simulink model "ConfiguredVirtualVehicleModel"  (R2023a)
settings: configuration reference "VehicleVariable" (kept outside this file)
StartFcn:
  | %tic
StopFcn:
  | %toc
undefined symbols (not defined in the file or in its folder): CtrlTcuInitGear, CtrlVcuCltch1InitCmd, Disabled, DriveCycleChoice, DriverPreviewDist, EnvAbsPrs, EnvAirTemp, EnvGrvty, EnvNomFrictionScaling, EnvNominalGrade, EnvWindVelX, EnvWindVelY, EnvWindVelZ, FTP75, PlntBattModNumCellSer, PlntBattNumMod, PlntBattTempInitDegC, PlntVehDstCGFrntAxl, PlntVehDstCGRearAxl, PlntVehInitLatPos, PlntVehInitLongPos, PlntVehInitPitchAng, PlntVehInitRollAng, PlntVehInitVertPos, PlntVehInitYawAng, PlntVehMass, PlntVehTrckWdth, PlntVehYawMomentInertia, ScnCRMaxLatAccel, ScnCRRadius, ScnDLCGateLongPos, ScnDLCLatRef, ScnDLCLatRefOffset, ScnDLCLongRefBpt, ScnDLCLongRefStartPos, ScnDLCVehicleWidth, ScnFHCounterDwellTime, ScnFHInitialDwellTime, ScnFHReturnTime, ScnFHRollRateZeroCross, ScnFHSteerAmp, ScnFHSteerSpeed, ScnISHandwheelRate, ScnISMaxHandwheelAng, ScnISMaxLatAccel, ScnISSteerHoldTime, ScnLongVelRef, ScnSDDwellTime, ScnSDSteerAmp, ScnSDSteerFreq, ScnSimTime, ScnSSFinalFreq, ScnSSSteerAmp, ScnSSSweepTime, ScnStartTime, ts
libraries: simulink x18, vehdynlibscenariocommon x7, autolibshared x5, vehdynlibviscommon x3, vehdynlibdriver x2, sim3dgroundtruthsensorlib x2, autolibsharedcommon x1, sharedtransform x1, sim3dlib x1, sim3dautolib x1
(part 4 of 5)

== system ConfiguredVirtualVehicleModel/Visualization/Vehicle XY Plotter/XY View Ref ==
  Bus Element In2 : Inport  PortName=VehFdbk
  Bus Element In1 : Inport  Port=2  PortName=Ref  Element=YRef
  Bus Element In3 : Inport  Port=2  PortName=Ref  Element=XRef
  Bus Selector1 : BusSelector  OutputSignals=Body.InertFrm.Cg.Ang.phi,Body.InertFrm.Cg.Ang.theta,Body.InertFrm.Cg.Ang.psi  OutputAsBus=on
  Bus Selector10 : BusSelector  OutputSignals=Wheels.Wheels.Fx,Wheels.Wheels.Fy
  Bus Selector5 : BusSelector  OutputSignals=Steering.Front.WhlAng.FL,Steering.Front.WhlAng.FR,Steering.Rear.WhlAng.RL,Steering.Rear.WhlAng.RR  OutputAsBus=on
  Bus Selector6 : BusSelector  OutputSignals=Body.InertFrm.Geom.Disp.X,Body.InertFrm.Geom.Disp.Y,Body.InertFrm.Geom.Disp.Z  OutputAsBus=on
  Bus Selector7 : BusSelector  OutputSignals=Body.InertFrm.Geom.Vel.Xdot,Body.InertFrm.Geom.Vel.Ydot,Body.InertFrm.Geom.Vel.Zdot  OutputAsBus=on
  Bus Selector9 : BusSelector  OutputSignals=Driveline.EngSpd,Driveline.TransInfo.TransInfo.Trans.TransGear  OutputAsBus=on
  Bus to Vector{,1..3} (4 alike) : BusToVector
  Ground1 : Ground
  Mux : Mux  Inputs=3
  Vehicle XY Plotter : vehdynlibviscommon/Vehicle XY Plot Configuration  extRef=on  extStats=on  extTireF=on  a=PlntVehDstCGFrntAxl  b=PlntVehDstCGRearAxl  w=PlntVehTrckWdth(1)  figBorder=10  bufferSize=1024  velNorm=5  tireFNorm=1000  pltDT=.1
  wires:
  Bus Selector7/1 -> Bus to Vector1/1
  Bus Selector5/1 -> Vehicle XY Plotter/4
  Ground1/1 -> Mux/3
  Bus Selector10/2 -> Vehicle XY Plotter/8  "<Fy>"
  Bus to Vector1/1 -> Vehicle XY Plotter/3
  Bus Selector10/1 -> Vehicle XY Plotter/7  "<Fx>"
  Bus Selector1/1 -> Bus to Vector2/1
  Bus Selector9/1 -> Bus to Vector3/1
  Bus Element In1/1 -> Mux/2
  Bus to Vector3/1 -> Vehicle XY Plotter/6
  Bus Element In3/1 -> Mux/1
  Mux/1 -> Vehicle XY Plotter/5
  Bus to Vector/1 -> Vehicle XY Plotter/1
  Bus Selector6/1 -> Bus to Vector/1
  Bus to Vector2/1 -> Vehicle XY Plotter/2
  Bus Element In2/1 -> Bus Selector10/1, Bus Selector9/1, Bus Selector5/1, Bus Selector7/1, Bus Selector1/1, Bus Selector6/1  "VehFdbk"

== system ConfiguredVirtualVehicleModel/Driver Commands/Driver Commands/Longitudinal Driver/Hill Hold ==
  LngRef : Inport
  <EnblDecelCmd> : Inport  Port=2
  <DecelOvrCmd> : Inport  Port=3
  <DecelHld> : Inport  Port=4
  <DecelZero> : Inport  Port=5
  Env : Inport  Port=6
  VehFdbk : Inport  Port=7
  Abs : Abs  ZeroCross=off  SaturateOnIntegerOverflow=off
  Abs1 : Abs  ZeroCross=off  SaturateOnIntegerOverflow=off
  Bus Selector : BusSelector  OutputSignals=Engine.EngSpdOut,Body.BdyFrm.Cg.Vel.xdot,Battery.BattSoc
  Bus Selector1 : BusSelector  OutputSignals=Body.BdyFrm.Cg.Vel.xdot
  Bus Selector2 : BusSelector  OutputSignals=Grade
  Compare To Constant : simulink/Logic and Bit Operations/Compare To Constant  relop=<=  const=.1  OutDataTypeStr=boolean  ZeroCross=off
  Compare To Constant1 : simulink/Logic and Bit Operations/Compare To Constant  relop=>=  const=.1  OutDataTypeStr=boolean  ZeroCross=off
  Compare To Constant2 : simulink/Logic and Bit Operations/Compare To Constant  relop=<=  const=500  OutDataTypeStr=boolean  ZeroCross=off
  Compare To Constant3 : simulink/Logic and Bit Operations/Compare To Constant  relop=<=  const=5  OutDataTypeStr=boolean  ZeroCross=off
  Compare To Constant4 : simulink/Logic and Bit Operations/Compare To Constant  relop=<=  const=.1  OutDataTypeStr=boolean  ZeroCross=off
  Data Type Conversion1 : DataTypeConversion  SaturateOnIntegerOverflow=off  RndMeth=Floor
  Igore Initialization Transients (t<=2s) : Subsystem
  Logical Operator : Logic  AllPortsSameDT=off  OutDataTypeStr=boolean
  Logical Operator1 : Logic  Inputs=3  AllPortsSameDT=off  OutDataTypeStr=boolean
  Logical Operator2 : Logic  Operator=OR  AllPortsSameDT=off  OutDataTypeStr=boolean
  Signal Specification : SignalSpecification  Unit=m/s
  Switch : Switch  Criteria=u2 > Threshold  SaturateOnIntegerOverflow=off  InputSameDT=off
  Switch1 : Switch  Criteria=u2 > Threshold  SaturateOnIntegerOverflow=off  InputSameDT=off
  Unit Conversion : UnitConversion
  VehFdbk1 : InportShadow  Port=7
  EnblDecelOvr : Outport
  DecelOvrCmd : Outport  Port=2
  DecelHld : Outport  Port=3
  DecelZero : Outport  Port=4
  VelFdbk : Outport  Port=5
  Grade : Outport  Port=6
  wires:
  Logical Operator2/1 -> Switch/3, Data Type Conversion1/1
  LngRef/1 -> Abs/1
  Abs/1 -> Compare To Constant/1
  Compare To Constant/1 -> Logical Operator/1
  Abs1/1 -> Compare To Constant1/1
  Compare To Constant1/1 -> Logical Operator/2
  Compare To Constant2/1 -> Logical Operator1/1
  Compare To Constant3/1 -> Logical Operator1/2
  Logical Operator1/1 -> Logical Operator2/1
  Logical Operator/1 -> Logical Operator2/2
  Compare To Constant4/1 -> Logical Operator1/3
  VehFdbk/1 -> Bus Selector/1
  Bus Selector/1 -> Compare To Constant2/1  "<EngSpdOut>"
  Bus Selector/2 -> Unit Conversion/1  "<xdot>"
  Bus Selector/3 -> Compare To Constant4/1  "<BattSoc>"
  Data Type Conversion1/1 -> Switch1/3
  <EnblDecelCmd>/1 -> Switch1/2, Switch/1, Switch/2
  Switch/1 -> EnblDecelOvr/1
  <DecelOvrCmd>/1 -> Switch1/1
  Switch1/1 -> DecelOvrCmd/1
  Env/1 -> Bus Selector2/1
  Bus Selector2/1 -> Grade/1, Abs1/1  "<Grade>"
  VehFdbk1/1 -> Bus Selector1/1
  Bus Selector1/1 -> Igore Initialization Transients (t<=2s)/1(<xdot>)  "<xdot>"
  Igore Initialization Transients (t<=2s)/1(VelFdbk) -> VelFdbk/1
  <DecelZero>/1 -> DecelZero/1
  <DecelHld>/1 -> DecelHld/1
  Unit Conversion/1 -> Signal Specification/1
  Signal Specification/1 -> Compare To Constant3/1

== system ConfiguredVirtualVehicleModel/Driver Commands/Driver Commands/Longitudinal Driver/Longitudinal Driver ==
  VelRef : Inport  Unit=m/s
  EnblAccelOvr : Inport  Port=2
  AccelOvrCmd : Inport  Port=3
  AccelHld : Inport  Port=4
  AccelZero : Inport  Port=5
  EnblDecelOvr : Inport  Port=6
  DecelOvrCmd : Inport  Port=7
  DecelHld : Inport  Port=8
  DecelZero : Inport  Port=9
  VelFdbk : Inport  Port=10  Unit=m/s
  Grade : Inport  Port=11
  ExtGearGround : Ground
  External Action Routing : Subsystem
  Longitudinal Driver : autolibsharedcommon/Longitudinal Driver  cntrlType=Predictive  shftType=None  vnom=vnom  Kp=Kp  Ki=Ki  Kaw=Kaw  Kff=Kff  Kg=Kg  tauerr=tauerr  tShift=tShift  tRev=tRev  tPark=tPark  pdlVec=pdlVec  upShftTbl=upShftTbl  dwnShftTbl=dwnShftTbl  GearInit=GearInit  tClutch=tClutch  VehVelVec=VehVelVec  KffVec=KffVec  KiVec=KiVec  KpVec=KpVec  KgVec=KgVec  m=m  Kpt=Kpt  Lvv=L  g=g  UpGearVec=UpGearVec  DownGearVec=DownGearVec  aMode=6  errUnit=m/s  aR=aR  bR=bR  cR=cR  tauPt=tauPt
      settings: LibrarySourceBlock=autolibshared/Longitudinal Driver/Longitudinal Driver
  Info : Outport  InitialOutput=0  VectorParamsAs1DForOutWhenUnconnected=off
  AccelCmd : Outport  Port=2  VectorParamsAs1DForOutWhenUnconnected=off
  DecelCmd : Outport  Port=3  VectorParamsAs1DForOutWhenUnconnected=off
  GearCmd : Outport  Port=4
  wires:
  VelRef/1 -> Longitudinal Driver/1
  VelFdbk/1 -> Longitudinal Driver/2
  Longitudinal Driver/1 -> Info/1
  Longitudinal Driver/2 -> AccelCmd/1
  Longitudinal Driver/3 -> DecelCmd/1
  Grade/1 -> Longitudinal Driver/3
  External Action Routing/1(ExtActions) -> Longitudinal Driver/5
  ExtGearGround/1 -> Longitudinal Driver/4
  Longitudinal Driver/4 -> GearCmd/1
  EnblAccelOvr/1 -> External Action Routing/1(EnblAccelOvr)
  AccelOvrCmd/1 -> External Action Routing/2(AccelOvrCmd)
  AccelHld/1 -> External Action Routing/3(AccelHld)
  AccelZero/1 -> External Action Routing/4(AccelZero)
  EnblDecelOvr/1 -> External Action Routing/5(EnblDecelOvr)
  DecelOvrCmd/1 -> External Action Routing/6(DecelOvrCmd)
  DecelHld/1 -> External Action Routing/7(DecelHld)
  DecelZero/1 -> External Action Routing/8(DecelZero)

== system ConfiguredVirtualVehicleModel/Driver Commands/Driver Commands/Predictive Driver/Hill Hold ==
  LngRef : Inport
  <EnblDecelCmd> : Inport  Port=2
  <DecelOvrCmd> : Inport  Port=3
  <DecelHld> : Inport  Port=4
  <DecelZero> : Inport  Port=5
  Env : Inport  Port=6
  VehFdbk : Inport  Port=7
  Abs : Abs  ZeroCross=off  SaturateOnIntegerOverflow=off
  Abs1 : Abs  ZeroCross=off  SaturateOnIntegerOverflow=off
  Bus Selector : BusSelector  OutputSignals=Engine.EngSpdOut,Body.BdyFrm.Cg.Vel.xdot,Battery.BattSoc
  Bus Selector1 : BusSelector  OutputSignals=Body.BdyFrm.Cg.Vel.xdot
  Bus Selector2 : BusSelector  OutputSignals=Grade
  Compare To Constant : simulink/Logic and Bit Operations/Compare To Constant  relop=<=  const=.1  OutDataTypeStr=boolean  ZeroCross=off
  Compare To Constant1 : simulink/Logic and Bit Operations/Compare To Constant  relop=>=  const=.1  OutDataTypeStr=boolean  ZeroCross=off
  Compare To Constant2 : simulink/Logic and Bit Operations/Compare To Constant  relop=<=  const=500  OutDataTypeStr=boolean  ZeroCross=off
  Compare To Constant3 : simulink/Logic and Bit Operations/Compare To Constant  relop=<=  const=5  OutDataTypeStr=boolean  ZeroCross=off
  Compare To Constant4 : simulink/Logic and Bit Operations/Compare To Constant  relop=<=  const=.1  OutDataTypeStr=boolean  ZeroCross=off
  Data Type Conversion1 : DataTypeConversion  SaturateOnIntegerOverflow=off  RndMeth=Floor
  Igore Initialization Transients (t<=2s) : Subsystem
  Logical Operator : Logic  AllPortsSameDT=off  OutDataTypeStr=boolean
  Logical Operator1 : Logic  Inputs=3  AllPortsSameDT=off  OutDataTypeStr=boolean
  Logical Operator2 : Logic  Operator=OR  AllPortsSameDT=off  OutDataTypeStr=boolean
  Signal Specification : SignalSpecification  Unit=m/s
  Switch : Switch  Criteria=u2 > Threshold  SaturateOnIntegerOverflow=off  InputSameDT=off
  Switch1 : Switch  Criteria=u2 > Threshold  SaturateOnIntegerOverflow=off  InputSameDT=off
  Unit Conversion : UnitConversion
  VehFdbk1 : InportShadow  Port=7
  EnblDecelOvr : Outport
  DecelOvrCmd : Outport  Port=2
  DecelHld : Outport  Port=3
  DecelZero : Outport  Port=4
  Grade : Outport  Port=5
  VelFdbk : Outport  Port=6
  wires:
  Logical Operator2/1 -> Switch/3, Data Type Conversion1/1
  LngRef/1 -> Abs/1
  Abs/1 -> Compare To Constant/1
  Compare To Constant/1 -> Logical Operator/1
  Abs1/1 -> Compare To Constant1/1
  Compare To Constant1/1 -> Logical Operator/2
  Compare To Constant2/1 -> Logical Operator1/1
  Compare To Constant3/1 -> Logical Operator1/2
  Logical Operator1/1 -> Logical Operator2/1
  Logical Operator/1 -> Logical Operator2/2
  Compare To Constant4/1 -> Logical Operator1/3
  VehFdbk/1 -> Bus Selector/1
  Bus Selector/1 -> Compare To Constant2/1  "<EngSpdOut>"
  Bus Selector/3 -> Compare To Constant4/1  "<BattSoc>"
  Data Type Conversion1/1 -> Switch1/3
  <EnblDecelCmd>/1 -> Switch1/2, Switch/1, Switch/2
  Switch/1 -> EnblDecelOvr/1
  <DecelOvrCmd>/1 -> Switch1/1
  Switch1/1 -> DecelOvrCmd/1
  Env/1 -> Bus Selector2/1
  Bus Selector2/1 -> Grade/1, Abs1/1  "<Grade>"
  VehFdbk1/1 -> Bus Selector1/1
  Bus Selector1/1 -> Igore Initialization Transients (t<=2s)/1(<xdot>)  "<xdot>"
  Igore Initialization Transients (t<=2s)/1(VelFdbk) -> VelFdbk/1
  <DecelZero>/1 -> DecelZero/1
  <DecelHld>/1 -> DecelHld/1
  Unit Conversion/1 -> Signal Specification/1
  Bus Selector/2 -> Unit Conversion/1  "<xdot>"
  Signal Specification/1 -> Compare To Constant3/1

== system ConfiguredVirtualVehicleModel/Driver Commands/Driver Commands/Predictive Stanley Driver/Hill Hold ==
  LngRef : Inport
  <EnblDecelCmd> : Inport  Port=2
  <DecelOvrCmd> : Inport  Port=3
  <DecelHld> : Inport  Port=4
  <DecelZero> : Inport  Port=5
  <CurvRef> : Inport  Port=6
  Env : Inport  Port=7
  VehFdbk : Inport  Port=8
  Abs : Abs  ZeroCross=off  SaturateOnIntegerOverflow=off
  Abs1 : Abs  ZeroCross=off  SaturateOnIntegerOverflow=off
  Bus Selector : BusSelector  OutputSignals=Engine.EngSpdOut,Body.BdyFrm.Cg.Vel.xdot,Battery.BattSoc
  Bus Selector1 : BusSelector  OutputSignals=Body.BdyFrm.Cg.Vel.xdot
  Bus Selector2 : BusSelector  OutputSignals=Grade
  Compare To Constant : simulink/Logic and Bit Operations/Compare To Constant  relop=<=  const=.1  OutDataTypeStr=boolean  ZeroCross=off
  Compare To Constant1 : simulink/Logic and Bit Operations/Compare To Constant  relop=>=  const=.1  OutDataTypeStr=boolean  ZeroCross=off
  Compare To Constant2 : simulink/Logic and Bit Operations/Compare To Constant  relop=<=  const=500  OutDataTypeStr=boolean  ZeroCross=off
  Compare To Constant3 : simulink/Logic and Bit Operations/Compare To Constant  relop=<=  const=5  OutDataTypeStr=boolean  ZeroCross=off
  Compare To Constant4 : simulink/Logic and Bit Operations/Compare To Constant  relop=<=  const=.1  OutDataTypeStr=boolean  ZeroCross=off
  Data Type Conversion1 : DataTypeConversion  SaturateOnIntegerOverflow=off  RndMeth=Floor
  Igore Initialization Transients (t<=2s) : Subsystem
  Logical Operator : Logic  AllPortsSameDT=off  OutDataTypeStr=boolean
  Logical Operator1 : Logic  Inputs=3  AllPortsSameDT=off  OutDataTypeStr=boolean
  Logical Operator2 : Logic  Operator=OR  AllPortsSameDT=off  OutDataTypeStr=boolean
  Signal Specification : SignalSpecification  Unit=m/s
  Switch : Switch  Criteria=u2 > Threshold  SaturateOnIntegerOverflow=off  InputSameDT=off
  Switch1 : Switch  Criteria=u2 > Threshold  SaturateOnIntegerOverflow=off  InputSameDT=off
  Unit Conversion : UnitConversion
  VehFdbk1 : InportShadow  Port=8
  EnblDecelOvr : Outport
  DecelOvrCmd : Outport  Port=2
  DecelHld : Outport  Port=3
  DecelZero : Outport  Port=4
  Grade : Outport  Port=5
  CurvRef : Outport  Port=6
  VelFdbk : Outport  Port=7
  wires:
  Signal Specification/1 -> Compare To Constant3/1
  Bus Selector/2 -> Unit Conversion/1  "<xdot>"
  Unit Conversion/1 -> Signal Specification/1
  <DecelHld>/1 -> DecelHld/1
  <DecelZero>/1 -> DecelZero/1
  VehFdbk1/1 -> Bus Selector1/1
  Bus Selector2/1 -> Abs1/1, Grade/1  "<Grade>"
  Env/1 -> Bus Selector2/1
  Switch1/1 -> DecelOvrCmd/1
  <DecelOvrCmd>/1 -> Switch1/1
  Switch/1 -> EnblDecelOvr/1
  <EnblDecelCmd>/1 -> Switch/2, Switch/1, Switch1/2
  Data Type Conversion1/1 -> Switch1/3
  Bus Selector/3 -> Compare To Constant4/1  "<BattSoc>"
  Bus Selector/1 -> Compare To Constant2/1  "<EngSpdOut>"
  VehFdbk/1 -> Bus Selector/1
  Compare To Constant4/1 -> Logical Operator1/3
  Logical Operator/1 -> Logical Operator2/2
  Logical Operator1/1 -> Logical Operator2/1
  Compare To Constant3/1 -> Logical Operator1/2
  Compare To Constant2/1 -> Logical Operator1/1
  Compare To Constant1/1 -> Logical Operator/2
  Abs1/1 -> Compare To Constant1/1
  Compare To Constant/1 -> Logical Operator/1
  Abs/1 -> Compare To Constant/1
  Logical Operator2/1 -> Data Type Conversion1/1, Switch/3
  <CurvRef>/1 -> CurvRef/1
  LngRef/1 -> Abs/1
  Bus Selector1/1 -> Igore Initialization Transients (t<=2s)/1(<xdot>)  "<xdot>"
  Igore Initialization Transients (t<=2s)/1(VelFdbk) -> VelFdbk/1

== system ConfiguredVirtualVehicleModel/Environment/Ground Feedback/3D Engine/3D Engine Source ==
  WheelFdbk : Inport
  Multiple Points : Subsystem  VariantControl=terrType==2
  Single Point : Subsystem  VariantControl=terrType ==1
  z : Outport
  DCM : Outport  Port=2

== system ConfiguredVirtualVehicleModel/Environment/Varying Friction/Varying Friction/Road Track Friction ==
  XWhl : Inport
  YWhl : Inport  Port=2
  Cg : Inport  Port=3
  2D Lookup Tbl for Scaling Fctr (Lambda) : Subsystem  TreatAsAtomicUnit=on
      mask init:
      | [~]=vehdynicon('vehdynblk',gcb);
  Bus Selector : BusSelector  OutputSignals=X,Y
  Cnst Lambda : Constant  Value=ones(4,1).*lambda_g
  Constant1 : Constant  Value=SplitLambdaTrck
  Creating Inertial Frm Bpt : Subsystem
  En at t = 0 : Subsystem
  "Lambda (t = 0) " : Memory  InitialCondition=ones(4,1).*lambda_g  InheritSampleTime=on
  Switch : Switch  Criteria=u2 > Threshold  SaturateOnIntegerOverflow=off  InputSameDT=off
  FricCoeffLambda : Outport
  wires:
  YWhl/1 -> 2D Lookup Tbl for Scaling Fctr (Lambda)/2(YWhl)
  XWhl/1 -> 2D Lookup Tbl for Scaling Fctr (Lambda)/1(XWhl)
  2D Lookup Tbl for Scaling Fctr (Lambda)/1(Lambda for each whl) -> Switch/1
  "Lambda (t = 0) "/1 -> FricCoeffLambda/1
  Switch/1 -> "Lambda (t = 0) "/1
  Cnst Lambda/1 -> Switch/3
  Constant1/1 -> Switch/2
  Cg/1 -> Bus Selector/1
  Creating Inertial Frm Bpt/1(XBpt) -> 2D Lookup Tbl for Scaling Fctr (Lambda)/3(XBpt)
  Creating Inertial Frm Bpt/2(YBpt) -> 2D Lookup Tbl for Scaling Fctr (Lambda)/4(YBpt)
  Bus Selector/1 -> Creating Inertial Frm Bpt/1(XCg)  "<X>"
  Bus Selector/2 -> Creating Inertial Frm Bpt/2(YCg)  "<Y>"
  En at t = 0/1(Out1) -> Creating Inertial Frm Bpt/Enable

== system ConfiguredVirtualVehicleModel/Environment/Varying Friction/Varying Friction/Wheel Coordinates ==
  FrntAxlLftX : Inport
  FrntAxlRghtX : Inport  Port=2
  RearAxlLftX : Inport  Port=3
  RearAxlRghtX : Inport  Port=4
  FrntAxlLftY : Inport  Port=5
  FrntAxlRghtY : Inport  Port=6
  RearAxlLftY : Inport  Port=7
  RearAxlRghtY : Inport  Port=8
  Matrix Concatenate : Concatenate  NumInputs=4  Mode=Multidimensional array
  Matrix Concatenate1 : Concatenate  NumInputs=4  Mode=Multidimensional array
  XWhl : Outport
  YWhl : Outport  Port=2
  wires:
  RearAxlRghtX/1 -> Matrix Concatenate/4
  Matrix Concatenate/1 -> XWhl/1
  RearAxlRghtY/1 -> Matrix Concatenate1/4
  RearAxlLftX/1 -> Matrix Concatenate/3
  RearAxlLftY/1 -> Matrix Concatenate1/3
  FrntAxlRghtX/1 -> Matrix Concatenate/2
  FrntAxlRghtY/1 -> Matrix Concatenate1/2
  FrntAxlLftY/1 -> Matrix Concatenate1/1
  FrntAxlLftX/1 -> Matrix Concatenate/1
  Matrix Concatenate1/1 -> YWhl/1

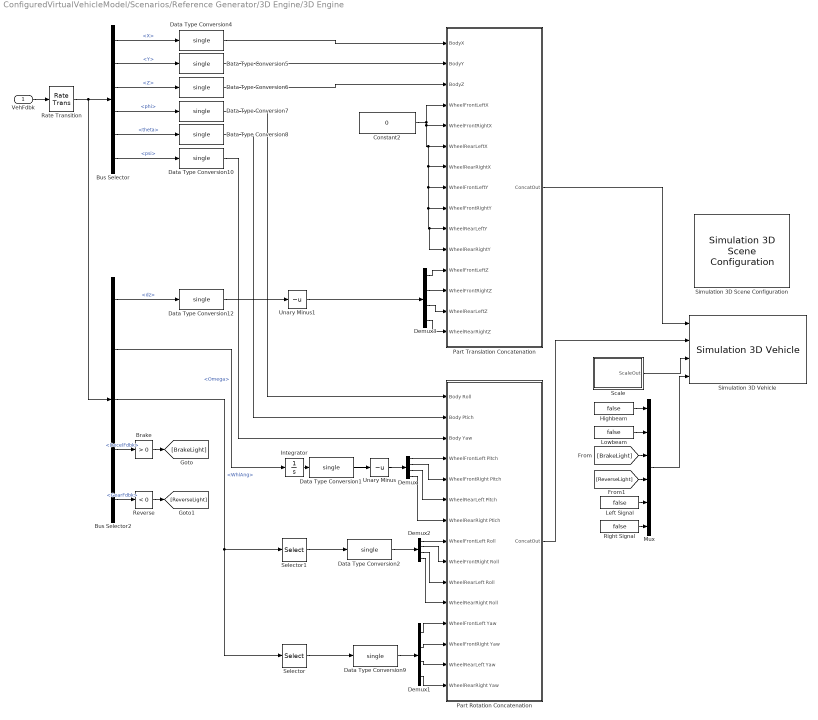
== system ConfiguredVirtualVehicleModel/Scenarios/Reference Generator/3D Engine/3D Engine ==
  VehFdbk : Inport
  Brake : simulink/Logic and Bit Operations/Compare To Constant  relop=>  const=0  OutDataTypeStr=boolean  ZeroCross=off
  Bus Selector : BusSelector  OutputSignals=Body.InertFrm.Geom.Disp.X,Body.InertFrm.Geom.Disp.Y,Body.InertFrm.Geom.Disp.Z,Body.InertFrm.Cg.Ang.phi,Body.InertFrm.Cg.Ang.theta,Body.InertFrm.Cg.Ang.psi
  Bus Selector2 : BusSelector  OutputSignals=Suspension.SuspWheel.dz,Wheels.Wheels.Omega,Suspension.SuspWheel.WhlAng,Driver.DecelFdbk,Driver.GearFdbk
  Constant2 : Constant  Value=0  OutDataTypeStr=single
  Data Type Conversion{1..2,4..10,12} (10 alike) : DataTypeConversion  OutDataTypeStr=single  SaturateOnIntegerOverflow=off  RndMeth=Floor
  Demux{,1..3} (4 alike) : Demux
  Highbeam : Constant  Value=false
  Integrator : Integrator  WrapState=on  WrappedStateUpperValue=2*pi  WrappedStateLowerValue=0  ZeroCross=off
  Left Signal : Constant  Value=false
  Lowbeam : Constant  Value=false
  Mux : Mux  Inputs=6
  Part Rotation Concatenation : Subsystem
  Part Translation Concatenation : Subsystem
  Rate Transition : RateTransition  OutPortSampleTime=dt3D
  Reverse : simulink/Logic and Bit Operations/Compare To Constant  relop=<  const=0  OutDataTypeStr=boolean  ZeroCross=off
  Right Signal : Constant  Value=false
  Scale : Subsystem
  Selector : Selector  NumberOfDimensions=2  InputPortWidth=3  IndexOptions=Index vector (dialog),Select all  Indices=[3],1  OutputSizes=1,1
  Selector1 : Selector  NumberOfDimensions=2  InputPortWidth=3  IndexOptions=Index vector (dialog),Select all  Indices=[1],1  OutputSizes=1,1
  Simulation 3D Scene Configuration : sim3dlib/Simulation 3D Scene Configuration  Priority=0  ProjectFormat=Default Scenes  SceneDesc=Open surface  ProjectName=C:\Program Files\MATLAB\R2023a\toolbox\shared\sim3d_projects\automotive_project\UE4\WindowsNoEditor\VehicleSimulation.exe  ScenePath=/Game/Maps/HwStrght  EnableOpenDRIVE=off  vehTagList={'Scene Origin'}  vehTag=Scene Origin  OpVisEn=off  Ts=dt3D  EnableWindow=on  EnableRemoteAccess=off  EnableWeather=off  SunAltitude=40.0  SunAzimuth=90  clouds=10  wind=1  fog=0  rain=0  EnableGeospatial=off  OriginHeight=200  OriginLatitude=40.744652  OriginLongitude=-73.988864  MapStyle=Aerial  AdditionalAssetIDs=[]  UseAdvancedSunSky=off  SolarTime=11  TimeZone=-5  Day=21  Month=9  Year=2022  UseDaylightSavingTime=on  DSTStartDay=10  DSTStartMonth=3  DSTEndDay=3  DSTEndMonth=11  DSTSwitchHour=2  sensorTag=MainCamera1  sensorId=1  sensorName=MainCamera1  mountLoc=Origin  offsetFlag=off  tmountOffset=[0, 0, 0]  rmountOffset=[0, 0, 0]  HorizontalResolution=1280  VerticalResolution=720  HorizontalFOV=60  mountPoint=[0 0 0]  mountOrientation=[0 0 0]  aMode=2  ID=1  GeoTrigger=Inactive
  Simulation 3D Vehicle : sim3dautolib/Simulation 3D Vehicle  Priority=-1  PassVehMesh=Muscle car  MeshPath=/MathWorksSimulation/Vehicles/Muscle/Meshes/SK_MuscleCar.SK_MuscleCar  VehColor=Red  ActorName=SimulinkVehicle1  VehLightsControl=on  HeadlightColor=[ 1, 1, 1 ]  HighBeamIntensity=100000  LowBeamIntensity=60000  HighBeamConeAngle=1.22  LowBeamConeAngle=1.22  LeftHeadlightOrientation=[ 0, 0 ]  RightHeadlightOrientation=[ 0, 0 ]  BrakelightIntensity=500  ReverselightIntensity=500  SignallightIntensity=500  SignallightPeriod=1  SignalPulseWidth=50  Translation=[PlntVehInitLongPos PlntVehInitLatPos -PlntVehInitVertPos; 0 0 0; 0 0 0; 0 0 0; 0 0 0]  Rotation=[PlntVehInitRollAng PlntVehInitPitchAng PlntVehInitYawAng; 0 0 0; 0 0 0; 0 0 0; 0 0 0]  Scale=ones( 5, 3 )  SampleTime=dt3D  ActorType=SimulinkVehicle  ID=1  aMode=2  ActorTag=SimulinkVehicle1
  Unary Minus : UnaryMinus
  Unary Minus1 : UnaryMinus
  wires:
  Unary Minus/1 -> Demux/1
  Unary Minus1/1 -> Demux3/1
  Selector1/1 -> Data Type Conversion2/1
  Selector/1 -> Data Type Conversion9/1
  Bus Selector2/5 -> Reverse/1  "<GearFdbk>"
  Bus Selector2/4 -> Brake/1  "<DecelFdbk>"
  Left Signal/1 -> Mux/5
  Right Signal/1 -> Mux/6
  Lowbeam/1 -> Mux/2
  [ReverseLight] -> Mux/4
  Reverse/1 -> [ReverseLight]
  Highbeam/1 -> Mux/1
  Brake/1 -> [BrakeLight]
  Mux/1 -> Simulation 3D Vehicle/4
  [BrakeLight] -> Mux/3
  Bus Selector/3 -> Data Type Conversion6/1  "<Z>"
  Bus Selector/5 -> Data Type Conversion8/1  "<theta>"
  Bus Selector/6 -> Data Type Conversion10/1  "<psi>"
  Bus Selector/2 -> Data Type Conversion5/1  "<Y>"
  Bus Selector/1 -> Data Type Conversion4/1  "<X>"
  Data Type Conversion7/1 -> Part Rotation Concatenation/1(Body Roll)
  Data Type Conversion4/1 -> Part Translation Concatenation/1(BodyX)
  Constant2/1 -> Part Translation Concatenation/4(WheelFrontLeftX), Part Translation Concatenation/11(WheelRearRightY), Part Translation Concatenation/10(WheelRearLeftY), Part Translation Concatenation/9(WheelFrontRightY), Part Translation Concatenation/8(WheelFrontLeftY), Part Translation Concatenation/7(WheelRearRightX), Part Translation Concatenation/6(WheelRearLeftX), Part Translation Concatenation/5(WheelFrontRightX)
  Data Type Conversion10/1 -> Part Rotation Concatenation/3(Body Yaw)
  Data Type Conversion5/1 -> Part Translation Concatenation/2(BodyY)
  Data Type Conversion8/1 -> Part Rotation Concatenation/2(Body Ptich)
  Data Type Conversion1/1 -> Unary Minus/1
  Integrator/1 -> Data Type Conversion1/1
  Demux1/2 -> Part Rotation Concatenation/13(WheelFrontRight Yaw)
  Demux1/1 -> Part Rotation Concatenation/12(WheelFrontLeft Yaw)
  Data Type Conversion9/1 -> Demux1/1
  Bus Selector2/2 -> Integrator/1  "<Omega>"
  Bus Selector2/3 -> Selector/1, Selector1/1  "<WhlAng>"
  Demux2/4 -> Part Rotation Concatenation/11(WheelRearRight Roll)
  Demux2/3 -> Part Rotation Concatenation/10(WheelRearLeft Roll)
  Demux2/2 -> Part Rotation Concatenation/9(WheelFrontRight Roll)
  Demux2/1 -> Part Rotation Concatenation/8(WheelFrontLeft Roll)
  Demux1/3 -> Part Rotation Concatenation/14(WheelRearLeft Yaw)
  Demux1/4 -> Part Rotation Concatenation/15(WheelRearRight Yaw)
  Data Type Conversion6/1 -> Part Translation Concatenation/3(BodyZ)
  VehFdbk/1 -> Rate Transition/1
  Demux3/2 -> Part Translation Concatenation/13(WheelFrontRightZ)
  Demux3/1 -> Part Translation Concatenation/12(WheelFrontLeftZ)
  Demux3/3 -> Part Translation Concatenation/14(WheelRearLeftZ)
  Demux3/4 -> Part Translation Concatenation/15(WheelRearRightZ)
  Data Type Conversion12/1 -> Unary Minus1/1
  Part Translation Concatenation/1(ConcatOut) -> Simulation 3D Vehicle/1
  Part Rotation Concatenation/1(ConcatOut) -> Simulation 3D Vehicle/2
  Bus Selector/4 -> Data Type Conversion7/1  "<phi>"
  Data Type Conversion2/1 -> Demux2/1
  Demux/1 -> Part Rotation Concatenation/4(WheelFrontLeft Pitch)
  Demux/2 -> Part Rotation Concatenation/5(WheelFrontRight Pitch)
  Demux/3 -> Part Rotation Concatenation/6(WheelRearLeft Pitch)
  Demux/4 -> Part Rotation Concatenation/7(WheelRearRight Ptich)
  Scale/1(ScaleOut) -> Simulation 3D Vehicle/3
  Rate Transition/1 -> Bus Selector2/1, Bus Selector/1
  Bus Selector2/1 -> Data Type Conversion12/1  "<dz>"

== system ConfiguredVirtualVehicleModel/Scenarios/Reference Generator/3D Engine/3D Engine Disabled ==
  VehFdbk : Inport
  Terminator : Terminator
  wires:
  VehFdbk/1 -> Terminator/1

== system ConfiguredVirtualVehicleModel/Scenarios/Reference Generator/Reference Generator/Braking ==
  "VehFdbk " : Inport
  Bus Creator : BusCreator  Inputs=3
  Bus Creator1 : BusCreator  Inputs=14
  Constant{,2..3,8} (4 alike) : Constant  Value=0
  Constant{1,4..7,9..12} (9 alike) : Constant  Value=false
  Ground : Ground
  Ground1 : Ground
  Ground2 : Ground
  Signal Specification : SignalSpecification  Unit=rad
  Signal Specification1 : SignalSpecification  Unit=one
  Signal Specification2 : SignalSpecification  Unit=one
  Straight Maneuver Reference Generator : vehdynlibscenariocommon/Straight Maneuver Reference Generator  t_start=.5  ax=0.5  xdot_r=20  xdotUnit=mph  brakingParam=Longitudinal displacement  t_brake=15  x_brake=200  ax_dec=1  BufferSize=40960  fixhw=on  faultTracking=on  xdot_rmax=1  xdot_rmean=2  r_max=1  hw_max=3  SimStopOnFault=off  aMode=2
  " Vis" : Outport
  " Ref" : Outport  Port=2
  " Fdbk" : Outport  Port=3
  wires:
  Straight Maneuver Reference Generator/1 -> Bus Creator1/1  "XRef"
  Ground/1 -> Bus Creator/1  "XRef"
  Ground2/1 -> Bus Creator/3  "ZRef"
  Constant6/1 -> Bus Creator1/7  "EnblAccelOvr"
  Constant/1 -> Bus Creator1/2  "LtrlRef"
  Bus Creator1/1 -> " Ref"/1
  Constant5/1 -> Bus Creator1/6  "SteerZero"
  Constant3/1 -> Signal Specification/1
  Constant7/1 -> Bus Creator1/9  "AccelHld"
  Signal Specification1/1 -> Bus Creator1/8  "AccelOvrCmd"
  Ground1/1 -> Bus Creator/2  "YRef"
  Signal Specification/1 -> Bus Creator1/4  "SteerOvrCmd"
  Bus Creator/1 -> " Vis"/1
  Constant12/1 -> Bus Creator1/14  "DecelZero"
  Constant1/1 -> Bus Creator1/3  "EnblSteerCmd"
  Constant10/1 -> Bus Creator1/11  "EnblDecelCmd"
  Constant11/1 -> Bus Creator1/13  "DecelHld"
  Signal Specification2/1 -> Bus Creator1/12  "DecelOvrCmd"
  Constant2/1 -> Signal Specification2/1
  Constant8/1 -> Signal Specification1/1
  Constant4/1 -> Bus Creator1/5  "SteerHld"
  Constant9/1 -> Bus Creator1/10  "AccelZero"
  "VehFdbk "/1 -> Straight Maneuver Reference Generator/1, " Fdbk"/1

== system ConfiguredVirtualVehicleModel/Scenarios/Reference Generator/Reference Generator/Double Lane Change ==
  "VehFdbk " : Inport
  Double Lane Change : vehdynlibscenariocommon/Lane Change Reference Generator  VariantControl=Variant1  ssMode=Initialize from model  ssVar=dlcSS35mph  t_start=t_start  XGate=XGate  xdot_r=xdot_r  xdotUnit=mph  xStart=xStart  vehW=vehW  latoff=latoff  lattoff=VEH.InitialLatPosition  centerSwitch=on  xSimStop=off  ssDefault=off  latRefbp=latRefbp  latRef=latRef  X_o=X_o  Y_o=Y_o  psi_o=phi_o  ssTol=1e-3  ssMaxTime=30  ssWSName=dlcSS35mph  aMode=2  use3DCones=off
      link override ISO 3888-2/Lateral Reference: LabelModeActiveChoice=1
  " Vis" : Outport  VectorParamsAs1DForOutWhenUnconnected=off
  " Ref" : Outport  Port=2  VectorParamsAs1DForOutWhenUnconnected=off
  " Fdbk" : Outport  Port=3  VectorParamsAs1DForOutWhenUnconnected=off
  wires:
  "VehFdbk "/1 -> " Fdbk"/1, Double Lane Change/1
  Double Lane Change/1 -> " Vis"/1
  Double Lane Change/2 -> " Ref"/1

== system ConfiguredVirtualVehicleModel/Scenarios/Reference Generator/Reference Generator/Drive Cycle ==
  "VehFdbk " : Inport
  Bus Creator : BusCreator  Inputs=3
  Bus Creator1 : BusCreator  Inputs=16
  Constant{,2..3,8,13..15,17} (8 alike) : Constant  Value=0
  Constant{1,4..7,9..12} (9 alike) : Constant  Value=false
  Constant16 : Constant  Value=zeros(1,3)
  Drive Cycle Source : autolibshared/Drive Cycle Source  cycleVar=FTP75  fileVar=L:\Bauto\matlab\test\toolbox\shared\autoblks\scenario\adac.txt  tfinal="2474  seconds"  cycleRepeat=off  outAccPort=off  outGearPort=off  gearList=No gear data  t_wot1=1  xdot_woto=0  xdot_wot1=26.8  t_wot2=30  xdot_wot2=0  t_wotend=40  srcUnit=m/s  outUnit=mph  srcAccUnit=m/s/s  outAccUnit=m/s^2  dt=0  aMode=6  faultOption=off  velBnd=2  velBndUnit=mph  inUnit=m/s  timeBnd=1  failOption=off  stopSim=off  maxFaultCnt=10  maxFaultTime=2  maxTotFaultTime=15  traceOption=off  dtTrace=1  traceWindow=10  lastDCname=FTP75  lastOutUnit=mph  lastDT=0  lastTB=1  lastSB=2  forceCalcBound=off
  Signal Specification : SignalSpecification  Unit=rad
  Signal Specification1 : SignalSpecification  Unit=one
  Signal Specification2 : SignalSpecification  Unit=one
  " Vis" : Outport  VectorParamsAs1DForOutWhenUnconnected=off
  " Ref" : Outport  Port=2  VectorParamsAs1DForOutWhenUnconnected=off
  " Fdbk" : Outport  Port=3  VectorParamsAs1DForOutWhenUnconnected=off
  wires:
  Constant2/1 -> Signal Specification2/1
  Constant8/1 -> Signal Specification1/1
  Constant4/1 -> Bus Creator1/7  "SteerHld"
  Signal Specification2/1 -> Bus Creator1/14  "DecelOvrCmd"
  Constant12/1 -> Bus Creator1/16  "DecelZero"
  Constant6/1 -> Bus Creator1/9  "EnblAccelOvr"
  Constant7/1 -> Bus Creator1/11  "AccelHld"
  Constant9/1 -> Bus Creator1/12  "AccelZero"
  Signal Specification1/1 -> Bus Creator1/10  "AccelOvrCmd"
  Constant11/1 -> Bus Creator1/15  "DecelHld"
  Constant10/1 -> Bus Creator1/13  "EnblDecelCmd"
  Constant5/1 -> Bus Creator1/8  "SteerZero"
  Signal Specification/1 -> Bus Creator1/6  "SteerOvrCmd"
  Constant3/1 -> Signal Specification/1
  Constant1/1 -> Bus Creator1/5  "EnblSteerCmd"
  Constant/1 -> Bus Creator1/2  "LtrlRef"
  Drive Cycle Source/1 -> Bus Creator1/1  "LngRef"
  Bus Creator1/1 -> " Ref"/1
  "VehFdbk "/1 -> " Fdbk"/1
  Bus Creator/1 -> " Vis"/1
  Constant15/1 -> Bus Creator/3  "ZRef"
  Constant14/1 -> Bus Creator/2  "YRef"
  Constant13/1 -> Bus Creator/1  "XRef"
  Constant16/1 -> Bus Creator1/3  "PoseRef"
  Constant17/1 -> Bus Creator1/4  "CurvRef"

== system ConfiguredVirtualVehicleModel/Scenarios/Reference Generator/Reference Generator/Fishhook ==
  "VehFdbk " : Inport
  Bus Creator : BusCreator  Inputs=3
  Constant : Constant  Value=0
  Constant1 : Constant  Value=0
  Constant2 : Constant  Value=0
  Fishhook : vehdynlibscenariocommon/Fishhook  ssMode=Initialize from model  ssVar=fh50mph  t_start=t_start  xdot_r=xdot_r  xdotUnit=mph  steerRate=steerRate  steerA=steerAFH  pFdbk=off  tDwell1=tDwell1  tDwell2=tDwell2  tSteer3=tSteer3  pZero=pZero  steerDir=off  ssDefault=off  X_o=0  Y_o=0  psi_o=0  ssTol=1  ssMaxTime=30  ssWSName=fh50mph  aMode=2
  " Vis" : Outport  VectorParamsAs1DForOutWhenUnconnected=off
  " Ref" : Outport  Port=2  VectorParamsAs1DForOutWhenUnconnected=off
  " Fdbk" : Outport  Port=3  VectorParamsAs1DForOutWhenUnconnected=off
  wires:
  Constant/1 -> Bus Creator/1  "XRef"
  Constant1/1 -> Bus Creator/2  "YRef"
  Constant2/1 -> Bus Creator/3  "ZRef"
  Bus Creator/1 -> " Vis"/1
  Fishhook/1 -> " Ref"/1
  "VehFdbk "/1 -> " Fdbk"/1, Fishhook/1

== system ConfiguredVirtualVehicleModel/Scenarios/Reference Generator/Reference Generator/Increasing Steer ==
  "VehFdbk " : Inport
  Bus Creator : BusCreator  Inputs=3
  Constant : Constant  Value=0
  Constant1 : Constant  Value=0
  Constant2 : Constant  Value=0
  Increasing Steer : vehdynlibscenariocommon/Slowly Increasing Steer  VariantControl=1  ssMode=Initialize from model  ssVar=is50mph  t_start=t_start  xdot_r=xdot_r  xdotUnit=mph  omega_hw=omega_hw  theta_max=theta_max  t_stop=t_stop  ay_max=ay_max  steerDir=off  ay_stop=on  ssDefault=off  X_o=0  Y_o=0  psi_o=0  ssTol=1  ssMaxTime=30  ssWSName=is50mph  aMode=2
  " Vis" : Outport  VectorParamsAs1DForOutWhenUnconnected=off
  " Ref" : Outport  Port=2  VectorParamsAs1DForOutWhenUnconnected=off
  " Fdbk" : Outport  Port=3  VectorParamsAs1DForOutWhenUnconnected=off
  wires:
  "VehFdbk "/1 -> " Fdbk"/1, Increasing Steer/1
  Bus Creator/1 -> " Vis"/1
  Increasing Steer/1 -> " Ref"/1  "LtrlRef"
  Constant2/1 -> Bus Creator/3  "ZRef"
  Constant1/1 -> Bus Creator/2  "YRef"
  Constant/1 -> Bus Creator/1  "XRef"

== system ConfiguredVirtualVehicleModel/Scenarios/Reference Generator/Reference Generator/Sine with Dwell ==
  "VehFdbk " : Inport
  Bus Creator : BusCreator  Inputs=3
  Constant : Constant  Value=0
  Constant1 : Constant  Value=0
  Constant2 : Constant  Value=0
  Sine With Dwell : vehdynlibscenariocommon/Sine With Dwell  VariantControl=3  ssMode=Initialize from model  ssVar=swd50mph  t_start=t_start  xdot_r=xdot_r  xdotUnit=mph  steerF=steerF  steerA=steerA  tdwell=tdwell  steerDir=off  ssDefault=off  X_o=0  Y_o=0  psi_o=0  ssTol=1  ssMaxTime=30  ssWSName=swd50mph  aMode=2
  " Vis" : Outport  VectorParamsAs1DForOutWhenUnconnected=off
  " Ref" : Outport  Port=2  VectorParamsAs1DForOutWhenUnconnected=off
  " Fdbk" : Outport  Port=3  VectorParamsAs1DForOutWhenUnconnected=off
  wires:
  Sine With Dwell/1 -> " Ref"/1
  "VehFdbk "/1 -> " Fdbk"/1, Sine With Dwell/1
  Bus Creator/1 -> " Vis"/1
  Constant2/1 -> Bus Creator/3  "ZRef"
  Constant1/1 -> Bus Creator/2  "YRef"
  Constant/1 -> Bus Creator/1  "XRef"

== system ConfiguredVirtualVehicleModel/Scenarios/Reference Generator/Reference Generator/Swept Sine ==
  "VehFdbk " : Inport
  Bus Creator : BusCreator  Inputs=3
  Constant : Constant  Value=0
  Constant1 : Constant  Value=0
  Constant2 : Constant  Value=0
  Swept Sine : vehdynlibscenariocommon/Swept Sine Reference Generator  VariantControl=2  ssMode=Initialize from model  ssVar=ss30mph  t_start=t_start  xdot_r=xdot_r  xdotUnit=mph  theta_hw=theta_hw  theta_hw_final=theta_hw_final  t_sweep=t_sweep  ssDefault=off  X_o=0  Y_o=0  psi_o=0  ssTol=1  ssMaxTime=30  ssWSName=ss30mph  aMode=2
  " Vis" : Outport  VectorParamsAs1DForOutWhenUnconnected=off
  " Ref" : Outport  Port=2  VectorParamsAs1DForOutWhenUnconnected=off
  " Fdbk" : Outport  Port=3  VectorParamsAs1DForOutWhenUnconnected=off
  wires:
  "VehFdbk "/1 -> " Fdbk"/1, Swept Sine/1
  Swept Sine/1 -> " Ref"/1
  Bus Creator/1 -> " Vis"/1
  Constant2/1 -> Bus Creator/3  "ZRef"
  Constant1/1 -> Bus Creator/2  "YRef"
  Constant/1 -> Bus Creator/1  "XRef"

== system ConfiguredVirtualVehicleModel/Vehicle/Trailer Input/Ground Info Trailer/Ground Info 2 AxleTrailer ==
  Env : Inport
  Bus Selector1 : BusSelector  OutputSignals=TraGnd.z.G_FL_z,TraGnd.z.G_FR_z,TraGnd.z.G_RL_z,TraGnd.z.G_RR_z
  Bus Selector3 : BusSelector  OutputSignals=Gnd.mu.mu_FL,Gnd.mu.mu_FR,Gnd.mu.mu_RL,Gnd.mu.mu_RR
  Vector Concatenate : Concatenate  NumInputs=4
  Vector Concatenate1 : Concatenate  NumInputs=4
  Ground : Outport
  Friction : Outport  Port=2
  wires:
  Bus Selector3/4 -> Vector Concatenate/4  "<mu_RR>"
  Bus Selector3/3 -> Vector Concatenate/3  "<mu_RL>"
  Bus Selector1/1 -> Vector Concatenate1/1  "<G_FL_z>"
  Bus Selector1/2 -> Vector Concatenate1/2  "<G_FR_z>"
  Bus Selector1/3 -> Vector Concatenate1/3  "<G_RL_z>"
  Bus Selector1/4 -> Vector Concatenate1/4  "<G_RR_z>"
  Bus Selector3/2 -> Vector Concatenate/2  "<mu_FR>"
  Bus Selector3/1 -> Vector Concatenate/1  "<mu_FL>"
  Vector Concatenate/1 -> Friction/1
  Vector Concatenate1/1 -> Ground/1
  Env/1 -> Bus Selector1/1, Bus Selector3/1

== system ConfiguredVirtualVehicleModel/Vehicle/Trailer Input/Ground Info Trailer/Ground Info 3 AxleTrailer ==
  Env : Inport
  Bus Selector1 : BusSelector  OutputSignals=TraGnd.z.G_FL_z,TraGnd.z.G_FR_z,TraGnd.z.G_RL_z,TraGnd.z.G_RR_z,TraGnd.z.G_RL_z,TraGnd.z.G_RR_z
  Bus Selector3 : BusSelector  OutputSignals=TraGnd.mu.mu_FL,TraGnd.mu.mu_FR,TraGnd.mu.mu_RL,TraGnd.mu.mu_RR,TraGnd.mu.mu_RL,TraGnd.mu.mu_RR
  Vector Concatenate : Concatenate  NumInputs=6
  Vector Concatenate1 : Concatenate  NumInputs=6
  Ground : Outport
  Friction : Outport  Port=2
  wires:
  Env/1 -> Bus Selector3/1, Bus Selector1/1
  Vector Concatenate1/1 -> Ground/1
  Vector Concatenate/1 -> Friction/1
  Bus Selector3/1 -> Vector Concatenate/1  "<mu_FL>"
  Bus Selector3/2 -> Vector Concatenate/2  "<mu_FR>"
  Bus Selector3/3 -> Vector Concatenate/3  "<mu_RL>"
  Bus Selector3/4 -> Vector Concatenate/4  "<mu_RR>"
  Bus Selector3/5 -> Vector Concatenate/5  "<mu_RL>"
  Bus Selector3/6 -> Vector Concatenate/6  "<mu_RR>"
  Bus Selector1/1 -> Vector Concatenate1/1  "<G_FL_z>"
  Bus Selector1/2 -> Vector Concatenate1/2  "<G_FR_z>"
  Bus Selector1/3 -> Vector Concatenate1/3  "<G_RL_z>"
  Bus Selector1/4 -> Vector Concatenate1/4  "<G_RR_z>"
  Bus Selector1/5 -> Vector Concatenate1/5  "<G_RL_z>"
  Bus Selector1/6 -> Vector Concatenate1/6  "<G_RR_z>"

== system ConfiguredVirtualVehicleModel/Driver Commands/Driver Commands/Longitudinal Driver/Hill Hold/Igore Initialization Transients (t<=2s) ==
  <xdot> : Inport
  Clock : Clock
  Dead Zone : DeadZone  ZeroCross=off
  Switch2 : Switch  Threshold=2  ZeroCross=off  SaturateOnIntegerOverflow=off  InputSameDT=off
  VelFdbk : Outport
  wires:
  Dead Zone/1 -> Switch2/3
  Clock/1 -> Switch2/2
  <xdot>/1 -> Dead Zone/1, Switch2/1
  Switch2/1 -> VelFdbk/1

== system ConfiguredVirtualVehicleModel/Driver Commands/Driver Commands/Longitudinal Driver/Longitudinal Driver/External Action Routing ==
  EnblAccelOvr : Inport  OutDataTypeStr=boolean  Unit=1  PortDimensions=1
  AccelOvrCmd : Inport  Port=2  OutDataTypeStr=double  Unit=1  PortDimensions=1
  AccelHld : Inport  Port=3  OutDataTypeStr=boolean  Unit=1  PortDimensions=1
  AccelZero : Inport  Port=4  OutDataTypeStr=boolean  Unit=1  PortDimensions=1
  EnblDecelOvr : Inport  Port=5  OutDataTypeStr=boolean  Unit=1  PortDimensions=1
  DecelOvrCmd : Inport  Port=6  OutDataTypeStr=double  Unit=1  PortDimensions=1
  DecelHld : Inport  Port=7  OutDataTypeStr=boolean  Unit=1  PortDimensions=1
  DecelZero : Inport  Port=8  OutDataTypeStr=boolean  Unit=1  PortDimensions=1
  Bus Creator2 : BusCreator  Inputs=8
  ExtActions : Outport
  wires:
  EnblAccelOvr/1 -> Bus Creator2/1  "EnblAccelOvr"
  AccelOvrCmd/1 -> Bus Creator2/2  "AccelOvrCmd"
  AccelHld/1 -> Bus Creator2/3  "AccelHld"
  AccelZero/1 -> Bus Creator2/4  "AccelZero"
  EnblDecelOvr/1 -> Bus Creator2/5  "EnblDecelOvr"
  DecelOvrCmd/1 -> Bus Creator2/6  "DecelOvrCmd"
  DecelHld/1 -> Bus Creator2/7  "DecelHld"
  DecelZero/1 -> Bus Creator2/8  "DecelZero"
  Bus Creator2/1 -> ExtActions/1  "ExtActions"

== system ConfiguredVirtualVehicleModel/Driver Commands/Driver Commands/Predictive Driver/Hill Hold/Igore Initialization Transients (t<=2s) ==
  <xdot> : Inport
  Clock : Clock
  Dead Zone : DeadZone  ZeroCross=off
  Switch2 : Switch  Threshold=2  ZeroCross=off  SaturateOnIntegerOverflow=off  InputSameDT=off
  VelFdbk : Outport
  wires:
  Dead Zone/1 -> Switch2/3
  Clock/1 -> Switch2/2
  <xdot>/1 -> Dead Zone/1, Switch2/1
  Switch2/1 -> VelFdbk/1

== system ConfiguredVirtualVehicleModel/Driver Commands/Driver Commands/Predictive Stanley Driver/Hill Hold/Igore Initialization Transients (t<=2s) ==
  <xdot> : Inport
  Clock : Clock
  Dead Zone : DeadZone  ZeroCross=off
  Switch2 : Switch  Threshold=2  ZeroCross=off  SaturateOnIntegerOverflow=off  InputSameDT=off
  VelFdbk : Outport
  wires:
  Dead Zone/1 -> Switch2/3
  Clock/1 -> Switch2/2
  <xdot>/1 -> Dead Zone/1, Switch2/1
  Switch2/1 -> VelFdbk/1
